simulink model "speed_t_S"  (R2019b)
settings: Solver=VariableStepAuto  StartTime=0.0  StopTime=10.0  RelTol=1e-3
settings Model: Creator=李瑾年  LastModifiedBy=李瑾年

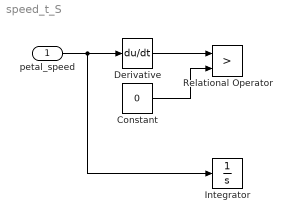
== system speed_t_S ==
  petal_speed : Inport
  Constant : Constant  Value=0
  Derivative : Derivative
  Integrator : Integrator
  Relational Operator : RelationalOperator  Operator=>  OutDataTypeStr=boolean  RndMeth=Simplest
  wires:
  petal_speed/1 -> Integrator/1, Derivative/1
  Derivative/1 -> Relational Operator/1
  Constant/1 -> Relational Operator/2
